simulink model "longi3"  (Simulink 8.6)
settings: Solver=ode4  SolverMode=SingleTasking  StartTime=0.0  StopTime=20  FixedStep=0.02  RelTol=1e-3  AbsTol=1e-6
values from neighbouring files (symbols this model uses):
  A = double(A)    [Script_BE_Mirage2000.m]
  B = [ M_dm ; Z_dm]    [Script_BE_Mirage2000.m]
  C = [0 , 1 ; 1 , 0 ; 0 , qbar*S_v0_Ref*Cza_0/(m*g)]    [Script_BE_Mirage2000.m]
  D = [0 ;0 ;qbar*S_v0_Ref*Cz_dm/(m*g)]    [Script_BE_Mirage2000.m]
libraries: simulink_extras x3, simulink x1
settings Model: Creator=scqdvfd  LastModifiedBy=5328100  ExtModeTrigMode=oneshot  ExtModeArmWhenConnect=off
settings DataIOCC: LimitDataPoints=off
settings OptimizationCC: BlockReduction=off  BooleanDataType=off  InitFltsAndDblsToZero=on
settings DebuggingCC: AlgebraicLoopMsg=none  SaveWithParameterizedLinksMsg=none  SignalResolutionControl=TryResolveAllWithWarning  SolverPrmCheckMsg=none  MultiTaskDSMMsg=warning  MultiTaskCondExecSysMsg=none  FcnCallInpInsideContextMsg=UseLocalSettings
settings HardwareCC: TargetUnknown=on
settings RTWCC: TemplateMakefile=grt_unix.tmf

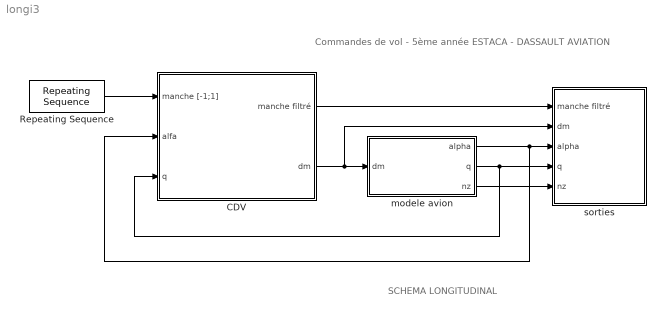
== system longi3 ==
  note: SCHEMA LONGITUDINAL
  note: Commandes de vol - 5ème année ESTACA - DASSAULT AVIATION
  CDV : Subsystem
  Repeating Sequence : simulink/Sources/Repeating Sequence  rep_seq_t=[0 2 2.1 12 12.1 100]  rep_seq_y=[0 0 -0.1 -0.1 0 0 ]
  modele avion : Subsystem
  sorties : Subsystem
  wires:
  modele avion/1(alpha) -> sorties/3(alpha), CDV/2(alfa)
  modele avion/2(q) -> sorties/4(q), CDV/3(q)
  modele avion/3(nz) -> sorties/5(nz)
  CDV/2(dm) -> sorties/2(dm), modele avion/1(dm)
  CDV/1(manche filtré) -> sorties/1(manche filtré)
  Repeating Sequence/1 -> CDV/1(manche [-1;1])

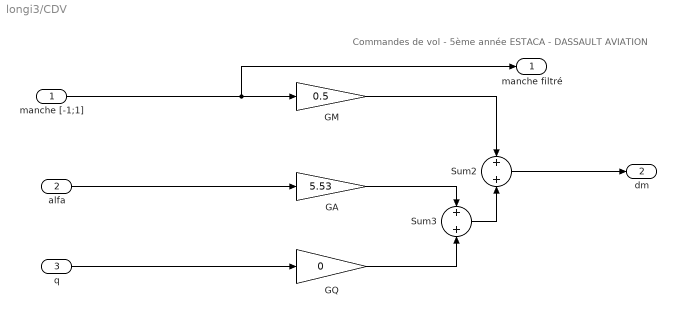
== system longi3/CDV ==
  note: Commandes de vol - 5ème année ESTACA - DASSAULT AVIATION
  manche [-1;1] : Inport
  alfa : Inport  Port=2
  q : Inport  Port=3
  GA : Gain  Gain=5.53  SaturateOnIntegerOverflow=on  OutDataTypeStr=Inherit: Same as input  ParamDataTypeStr=Inherit: Same as input
  GM : Gain  Gain=0.5  SaturateOnIntegerOverflow=on  OutDataTypeStr=Inherit: Same as input  ParamDataTypeStr=Inherit: Same as input
  GQ : Gain  Gain=0  SaturateOnIntegerOverflow=on  OutDataTypeStr=Inherit: Same as input  ParamDataTypeStr=Inherit: Same as input
  Sum2 : Sum  SaturateOnIntegerOverflow=on  InputSameDT=on  OutDataTypeStr=Inherit: Same as first input
  Sum3 : Sum  SaturateOnIntegerOverflow=on  InputSameDT=on  OutDataTypeStr=Inherit: Same as first input
  manche filtré : Outport  InitialOutput=0
  dm : Outport  Port=2  InitialOutput=0
  wires:
  GM/1 -> Sum2/1
  Sum2/1 -> dm/1
  q/1 -> GQ/1
  GA/1 -> Sum3/1
  GQ/1 -> Sum3/2
  Sum3/1 -> Sum2/2
  manche [-1;1]/1 -> manche filtré/1, GM/1
  alfa/1 -> GA/1

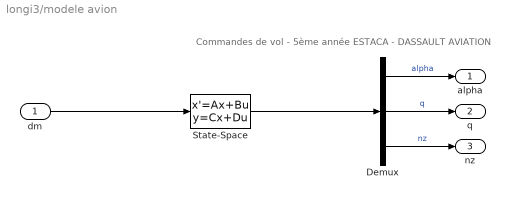
== system longi3/modele avion ==
  note: Commandes de vol - 5ème année ESTACA - DASSAULT AVIATION
  dm : Inport
  Demux : Demux  Outputs=3
  State-Space : StateSpace  A=A  B=B  C=C  D=D  X0=0
  alpha : Outport  InitialOutput=0
  q : Outport  Port=2  InitialOutput=0
  nz : Outport  Port=3  InitialOutput=0
  wires:
  Demux/3 -> nz/1  "nz"
  Demux/2 -> q/1  "q"
  Demux/1 -> alpha/1  "alpha"
  dm/1 -> State-Space/1
  State-Space/1 -> Demux/1

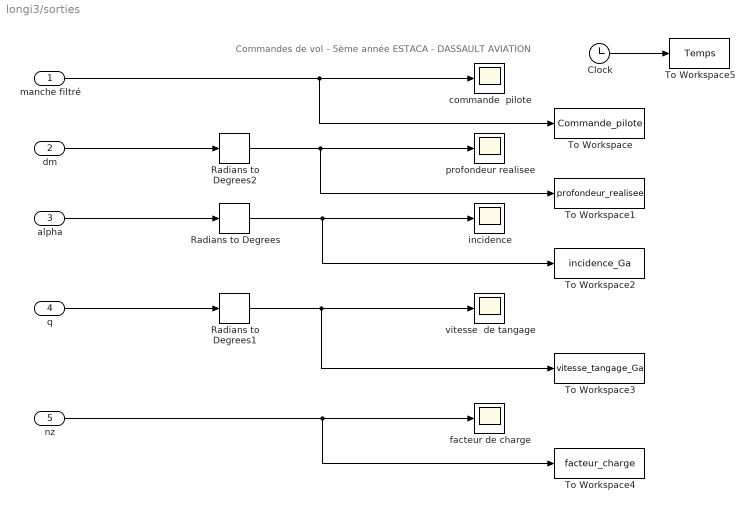
== system longi3/sorties ==
  note: Commandes de vol - 5ème année ESTACA - DASSAULT AVIATION
  manche filtré : Inport
  dm : Inport  Port=2
  alpha : Inport  Port=3
  q : Inport  Port=4
  nz : Inport  Port=5
  Clock : Clock
  Radians to Degrees : simulink_extras/Transformations/Radians to Degrees
  Radians to Degrees1 : simulink_extras/Transformations/Radians to Degrees
  Radians to Degrees2 : simulink_extras/Transformations/Radians to Degrees
  To Workspace : ToWorkspace  VariableName=Commande_pilote  SampleTime=-1
  To Workspace1 : ToWorkspace  VariableName=profondeur_realisee  SampleTime=-1
  To Workspace2 : ToWorkspace  VariableName=incidence_Ga  SampleTime=-1
  To Workspace3 : ToWorkspace  VariableName=vitesse_tangage_Ga  SampleTime=-1
  To Workspace4 : ToWorkspace  VariableName=facteur_charge  SampleTime=-1
  To Workspace5 : ToWorkspace  VariableName=Temps  SampleTime=-1
  commande  pilote : Scope
  facteur de charge : Scope
  incidence : Scope
  profondeur realisee : Scope
  vitesse  de tangage : Scope
  wires:
  manche filtré/1 -> To Workspace/1, commande  pilote/1
  dm/1 -> Radians to Degrees2/1
  alpha/1 -> Radians to Degrees/1
  q/1 -> Radians to Degrees1/1
  nz/1 -> To Workspace4/1, facteur de charge/1
  Radians to Degrees2/1 -> To Workspace1/1, profondeur realisee/1
  Radians to Degrees/1 -> To Workspace2/1, incidence/1
  Radians to Degrees1/1 -> To Workspace3/1, vitesse  de tangage/1
  Clock/1 -> To Workspace5/1
